simulink model "HIL_Testing_SW"  (Simulink 7.5)
settings: Solver=ode1  StartTime=0.0  StopTime=Inf  FixedStep=0.001  RelTol=1e-3
PostLoadFcn:
  | , if any(exist('dsrtsu_mdlpostloadfcn', 'file') == [2, 3, 6]), try dsrtsu_mdlpostloadfcn('Execute', bdroot); catch fprintf('Error in PostLoadFcn (dsrtsu_mdlpostloadfcn) for model "%s":\n %s\n', bdroot, lasterr); end, end,
undefined symbols (not defined in the file): CeBSER_Cnt_NumTempAxisPts, ChargeCord, ChargeCord_Control, ChargeToSOCCurr, ChrgCurrLim, CrntSens1Fine, CS_SOCSetPt, CyclerMaxChrgPwr, CyclerMaxDschrgPwr, deltaAhr, Drive_1, Drive_10, Drive_11, Drive_12, Drive_13, Drive_14, Drive_15, Drive_16, Drive_17, Drive_18, Drive_19, Drive_2, Drive_20, Drive_21, Drive_22, Drive_23, Drive_24, Drive_25, Drive_26, Drive_27, Drive_28, Drive_29, Drive_3, Drive_30, Drive_31, Drive_32, Drive_33, Drive_34, Drive_35, Drive_36, Drive_37, Drive_38, Drive_39, Drive_4, Drive_40, Drive_41, Drive_42, Drive_43, Drive_44, Drive_45, Drive_46, Drive_47, Drive_48, Drive_49, Drive_5, Drive_50, Drive_51, Drive_6, Drive_7, Drive_8 ... (+50)
libraries: simulink x129, rtican x50, rti2211sailib x5, rti2211serlib x5, rti2202miolib x3
(part 15 of 23)

== system HIL_Testing_SW/TX/Chiller/ChillerCmndTxDecision/ChillerCommands ==
  ReadChillerSP : Constant  Value=[82 83 13 13 13 13 13 13]  OutDataTypeMode=uint8  OutDataType=fixdt(1, 16)  OutScaling=2^0  OutDataTypeStr=uint8
  ReadChillerStatus : Constant  Value=[82 87 13 13 13 13 13 13]  OutDataTypeMode=uint8  OutDataType=fixdt(1, 16)  OutScaling=2^0  OutDataTypeStr=uint8
  ReadChillerTemp : Constant  Value=[82 84 13 13 13 13 13 13]  OutDataTypeMode=uint8  OutDataType=fixdt(1, 16)  OutScaling=2^0  OutDataTypeStr=uint8
  SetEchoOn : Constant  Value=[83 69 49 13 13 13 13 13]  OutDataTypeMode=uint8  OutDataType=fixdt(1, 16)  OutScaling=2^0  OutDataTypeStr=uint8
  TurnChillerOff : Constant  Value=[83 79 48 13 13 13 13 13]  OutDataTypeMode=uint8  OutDataType=fixdt(1, 16)  OutScaling=2^0  OutDataTypeStr=uint8
  TurnChillerOn : Constant  Value=[83 79 49 13 13 13 13 13]  OutDataTypeMode=uint8  OutDataType=fixdt(1, 16)  OutScaling=2^0  OutDataTypeStr=uint8
  TurnChiller_On : Outport
  TurnChiller_Off : Outport  Port=2
  SetEcho_On : Outport  Port=3
  ReadChiller_Status : Outport  Port=4
  ReadChillerSetPoint : Outport  Port=5
  ReadChiller_Temp : Outport  Port=6
  wires:
  TurnChillerOn/1 -> TurnChiller_On/1  "TurnChiller_On"
  TurnChillerOff/1 -> TurnChiller_Off/1  "TurnChiller_Off"
  SetEchoOn/1 -> SetEcho_On/1  "SetEcho_On"
  ReadChillerStatus/1 -> ReadChiller_Status/1  "ReadChiller_Status"
  ReadChillerSP/1 -> ReadChillerSetPoint/1  "ReadChillerSetPoint"
  ReadChillerTemp/1 -> ReadChiller_Temp/1  "ReadChiller_Temp"

== system HIL_Testing_SW/TX/Chiller/ChillerCmndTxDecision/ChillerRxProcessing ==
  RxBytes : Inport  OutDataType=fixdt(1, 16)  OutScaling=2^0
  NumRxBytes : Inport  Port=2  OutDataType=fixdt(1, 16)  OutScaling=2^0
  WaitRx : Inport  Port=3  OutDataType=fixdt(1, 16)  OutScaling=2^0
  ReadChillerStatus_Action : Inport  Port=4  OutDataType=fixdt(1, 16)  OutScaling=2^0
  ReadChillerSP_Action : Inport  Port=5  OutDataType=fixdt(1, 16)  OutScaling=2^0
  ReadChillerTemp_Action : Inport  Port=6  OutDataType=fixdt(1, 16)  OutScaling=2^0
  ChillerPositiveResponse : Subsystem
  ChillerStatus : Subsystem
  If : If  NumInputs=4  IfExpression=u1 == 1  ElseIfExpressions=u2 == 1, u3 == 1, u4 ==1
  ReadChillerSP : Subsystem  TreatAsAtomicUnit=on
  ReadChillerTemp : Subsystem
  RxChillerByteShifter : Subsystem
  Terminator : Terminator
  Terminator1 : Terminator
  Terminator2 : Terminator
  ChillerPosResponse : Outport  OutDataType=fixdt(1, 16)  OutScaling=2^0
  ChillerOn : Outport  Port=2  OutDataType=fixdt(1, 16)  OutScaling=2^0
  wires:
  RxBytes/1 -> RxChillerByteShifter/1(RxChillerBytes)
  ReadChillerSP/1(RxReadChillerSetPoint) -> Terminator/1
  ReadChillerTemp/1(RxReadChillerTemp) -> Terminator1/1
  If/1 -> ReadChillerSP/Action
  If/2 -> ReadChillerTemp/Action
  NumRxBytes/1 -> [NumRxBytes], RxChillerByteShifter/2(NumRxBytes)
  [NumRxBytes] -> ReadChillerSP/1(NumRxBytes)
  [NumRxBytes] -> ReadChillerTemp/1(NumRxBytes)
  If/5 -> Terminator2/1
  ChillerPositiveResponse/1(ChillerPositiveResponse) -> ChillerPosResponse/1
  WaitRx/1 -> If/3
  ReadChillerStatus_Action/1 -> If/4
  If/4 -> ChillerStatus/Action
  ChillerStatus/1(ChillerOn) -> ChillerOn/1
  If/3 -> ChillerPositiveResponse/Action
  ReadChillerTemp_Action/1 -> If/2
  ReadChillerSP_Action/1 -> If/1

== system HIL_Testing_SW/TX/Chiller/ChillerCmndTxDecision/CreateChillerSPCmnd ==
  ChillerT_SP : Inport  OutDataType=fixdt(1, 16)  OutScaling=2^0
  ChillerMux : Mux  Inputs=8
      settings: DisplayOption=signals
  DeMuxChillerInputNumber : Subsystem
  SetChillerSPCmnd : Outport  OutDataType=fixdt(1, 16)  OutScaling=2^0
  wires:
  ChillerT_SP/1 -> DeMuxChillerInputNumber/1(ChillerSP_Number)
  DeMuxChillerInputNumber/4(OnesDigitAscii) -> ChillerMux/5
  DeMuxChillerInputNumber/6(TenthsDigitAscii) -> ChillerMux/7
  ChillerMux/1 -> SetChillerSPCmnd/1
  DeMuxChillerInputNumber/2(PosOrNegAscii) -> ChillerMux/3
  DeMuxChillerInputNumber/3(TensDigitAscii) -> ChillerMux/4
  DeMuxChillerInputNumber/1(Ascii_S) -> ChillerMux/1, ChillerMux/2
  DeMuxChillerInputNumber/5(Ascii_Pt) -> ChillerMux/6
  DeMuxChillerInputNumber/7(Ascii_CarriageReturn) -> ChillerMux/8

== system HIL_Testing_SW/TX/Chiller/ChillerCmndTxDecision/CreateChillerSPCmnd2 ==
  ChillerT_SP : Inport  OutDataType=fixdt(1, 16)  OutScaling=2^0
  ChillerMux : Mux  Inputs=8
      settings: DisplayOption=signals
  DeMuxChillerInputNumber : Subsystem
  Gain : Gain  ParameterDataType=fixdt(1, 16)  ParameterScaling=2^0  OutDataTypeMode=uint8  OutDataType=fixdt(1, 16)  OutScaling=2^0  OutDataTypeStr=uint8
  SetChillerSPCmnd : Outport  OutDataType=fixdt(1, 16)  OutScaling=2^0
  wires:
  DeMuxChillerInputNumber/7(Ascii_CarriageReturn) -> ChillerMux/8
  DeMuxChillerInputNumber/5(Ascii_Pt) -> ChillerMux/6
  DeMuxChillerInputNumber/1(Ascii_S) -> ChillerMux/2, ChillerMux/1
  DeMuxChillerInputNumber/3(TensDigitAscii) -> ChillerMux/4
  DeMuxChillerInputNumber/2(PosOrNegAscii) -> ChillerMux/3
  ChillerMux/1 -> Gain/1
  DeMuxChillerInputNumber/6(TenthsDigitAscii) -> ChillerMux/7
  DeMuxChillerInputNumber/4(OnesDigitAscii) -> ChillerMux/5
  ChillerT_SP/1 -> DeMuxChillerInputNumber/1(ChillerSP_Number)
  Gain/1 -> SetChillerSPCmnd/1

== system HIL_Testing_SW/TX/TX PTEI/Tx_Contactor_Msg/msg_0x186 ==
  Ignition : Inport  OutDataType=fixdt(1, 16)  OutScaling=2^0
  InvVoltatge : Inport  Port=2  OutDataType=fixdt(1, 16)  OutScaling=2^0
  Trigger : TriggerPort  TriggerType=function-call
  ContactorsClosed1 : Constant  OutDataType=sfix(16)  OutScaling=2^0  OutDataTypeStr=Inherit: Inherit via back propagation
  ContactorsClosed4 : Constant  Value=0  OutDataType=sfix(16)  OutScaling=2^0  OutDataTypeStr=Inherit: Inherit via back propagation
  Ground_{1..16} (16 alike) : Ground
  PTEI_Hybrid_Status_1 : rtican/RTICAN Transmit (TX)   SystemSampleTime=-1  Reserved1=[]  Reserved2=[]  Reserved3=[]  Reserved4=[]  SfcnMessage=[]  Msg_Struct=[]  BoardTypeNo=[]  BoardNo=[]  ChannelNo=[]  Parameters=[]  DialogFcn=[]  UnitName=[]  Revision=[]  UnitValues=[]  DSProperties=struct('RTI',struct('Version',uint32(5),'BlockType',struct('isSLSource',uint8(1),'isSLSink',uint8(1),'isHWSource',uint8(0),'isHWSink',uint8(0),'isSetup',uint8(0),'isInline',uint8(1),'isNonInline',uint8(0),'isInterrupt',uint8(0),'isChannelwise',uint8(0)),'IOBoardType','RTICAN','UnitType','MESSAGE','Identifier','TX','DialogType','MSVC','BlockSet','RTICAN','SlaveProcessor','CAN'))  RTIBlockInterface=struct('InputPortsWidth',int32([1 1 1 1 1 1 1 1 1 1 1 1 1 1 1 1 1 1 1]),'InputPortsActive',[1 1 1 1 1 1 1 1 1 1 1 1 1 1 1 1 1 1 1],'InputPortsName',{{'RdHVInvRatVlt','HybCrpCstCrvRq','EstMtrPwrLoss','HybGrdBrkgAct','TransFldPmpMtrDrtd','EngActDmpgDsblReq','HybACCompRq','EstMtrPwrLossV','HybExtndDcFuelCORq','HybCmmdEngTrqLmtd','HESSI_EngStrtTyp','HESSI_EngStrtStpMd','HybCrnkAbrtd','CnvntlEngStrtEnbld','RdPTHVCntrReq','HybCmmFailRdPwrCmd','HybRdcdTrqCapMd1Cmnd','HybDFCOReq','RdHVInvRatVltV'}},'InputPortsDataType',{{'SS_DOUBLE','SS_DOUBLE','SS_DOUBLE','SS_DOUBLE','SS_DOUBLE','SS_DOUBLE','SS_DOUBLE','SS_DOUBLE','SS_DOUBLE','SS_DOUBLE','SS_DOUBLE','SS_DOUBLE','SS_DOUBLE','SS_DOUBLE','SS_DOUBLE','SS_DOUBLE','SS_DOUBLE','SS_DOUBLE','SS_DOUBLE'}},'OutputPortsWidth',int32(0),'OutputPortsActive',0,'OutputPortsName',{{''}},'DialogFcn','rtican_message_interface_gui','BlockDisplay',{{'','center'}},'IconTransparency','on','InitLevel',3,'BlockName',struct('Token',{{'PTEI_Hybrid_Status_1'}}),'SampleTime',{{-1}},'TriggerPort',{{'none'}},'EnablePort',{{'none'}})  RTIBlockParameters=struct('BoardTypeNo',{{4302,'OFF',[]}},'BoardNo',{{1,'ON',[1 16]}},'ChannelNo',{{1,'ON',[1 4]}},'Parameters',{{struct('DataFileSupport',struct('DataFileSelectedMaster',1,'DataFileSelectedLocal',1,'DataFileName',['c:\data\databases\8.4.5 (140425)\globala - hs.dbc|'],'DataFileDate',{{{['24-Apr-2014 15:37:04']}}},'SelectedFile',['..\databases\8.4.5 (140425)\globala - hs.dbc'],'InterfaceFcn','rtican_dbc_file_parser'),'Options',struct('StatusSelected',0,'TimeSelected',0,'DeltaTimeSelected',0,'DelayTimeSelected',0,'DelayTimeTXCommandSelected',0,'EncodeSetUnusedBitsToOne',0,'EnableMsgLoopback',0,'TriggerPort',struct('Selected',0,'TriggerType',0),'EnablePortSelected',0,'SignalOnPortnameSelected',1,'UserCoding',struct('Selected',0,'InterfaceFile','UserEncodingFile','FcnName','UserEncodeFcn','InportSelected',0,'InportWidth',1,'OutportSelected',0,'OutportWidth',1),'TerminationMsg',struct('Selected',0,'Byte0_7','0'),'InitialMsg',struct('Selected',0,'Byte0_7','0')),'Message',struct('MsgOnBlocknameSelected',1,'MsgName','PTEI_Hybrid_Status_1','MsgIdFormat',0,'MsgId',390,'MsgLength',7,'NumSignals',19,'SampleTime',-1,'StartTime',struct('Selected',0,'Value',0),'AutoRepeatTime',struct('Selected',0,'Value',0.1),'Timeout',struct('Selected',0,'Value',0.1),'DelayTime',struct('Selected',0,'Value',0.1),'Signal',struct('SgnName',{'RdHVInvRatVlt','HybCrpCstCrvRq','EstMtrPwrLoss','HybGrdBrkgAct','TransFldPmpMtrDrtd','EngActDmpgDsblReq','HybACCompRq','EstMtrPwrLossV','HybExtndDcFuelCORq','HybCmmdEngTrqLmtd','HESSI_EngStrtTyp','HESSI_EngStrtStpMd','HybCrnkAbrtd','CnvntlEngStrtEnbld','RdPTHVCntrReq','HybCmmFailRdPwrCmd','HybRdcdTrqCapMd1Cmnd','HybDFCOReq','RdHVInvRatVltV'},'SgnStartBit',{0,9,16,25,26,27,28,30,31,32,40,44,48,49,50,52,53,54,55},'SgnLength',{9,3,8,1,1,1,2,1,1,8,4,4,1,1,2,1,1,1,1},'SgnType',{0,0,0,0,0,0,0,0,0,0,0,0,0,0,0,0,0,0,0},'ModeValue',{-1,-1,-1,-1,-1,-1,-1,-1,-1,-1,-1,-1,-1,-1,-1,-1,-1,-1,-1},'DataType',{0,0,0,0,0,0,0,0,0,0,0,0,0,0,0,0,0,0,0},'ByteLayout',{2,2,2,2,2,2,2,2,2,2,2,2,2,2,2,2,2,2,2},'Factor',{1,1,0.25,1,1,1,1,1,1,0.75,1,1,1,1,1,1,1,1,1},'Offset',{0,0,0,0,0,0,0,0,0,-90,0,0,0,0,0,0,0,0,0},'SgnComment',{{''},{''},{''},{''},{''},{''},{''},{''},{''},{''},{''},{''},{''},{''},{''},{''},{''},{['DFCO = Deceleration Fuel Cut Off']},{''}},'SgnUnit',{'volts','','kW','','','','','','','Nm','','','','','','','','',''},'Min',{0,0,0,0,0,0,0,0,0,-90,0,0,0,0,0,0,0,0,0},'Max',{511,7,63.75,1,1,1,3,1,1,101.25,15,15,1,1,3,1,1,1,1},'SLDataType',{'SS_DOUBLE','SS_DOUBLE','SS_DOUBLE','SS_DOUBLE','SS_DOUBLE','SS_DOUBLE','SS_DOUBLE','SS_DOUBLE','SS_DOUBLE','SS_DOUBLE','SS_DOUBLE','SS_DOUBLE','SS_DOUBLE','SS_DOUBLE','SS_DOUBLE','SS_DOUBLE','SS_DOUBLE','SS_DOUBLE','SS_DOUBLE'}),'MsgIdNumFormat',0,'MsgComment',{{''}}),'Version',1.2,'general',struct('isFromLib',0)),'OFF',[]}},'GroupId',{{struct('Group',{{'RTICAN'}},'No',8,'Behavior',{{'NAMECHANGE'}},'BlockType',{{'SINK'}},'NameChangeFlag',0),'OFF',[]}},'SFcnRTICANMessage',{{struct('MsgType','TX','SFcnPortType','Scalar','MsgName','PTEI_Hybrid_Status_1','MsgIdFormat','STD','MsgId',390,'MsgLength',7,'NumSignals',19,'SampleTime',-1,'StartTime',struct('Selected','no','Value',0),'AutoRepeatTime',struct('Selected','no','Value',0.1),'Timeout',struct('Selected','no','Value',0.1),'Signal',struct('SgnName',{'RdHVInvRatVlt','HybCrpCstCrvRq','EstMtrPwrLoss','HybGrdBrkgAct','TransFldPmpMtrDrtd','EngActDmpgDsblReq','HybACCompRq','EstMtrPwrLossV','HybExtndDcFuelCORq','HybCmmdEngTrqLmtd','HESSI_EngStrtTyp','HESSI_EngStrtStpMd','HybCrnkAbrtd','CnvntlEngStrtEnbld','RdPTHVCntrReq','HybCmmFailRdPwrCmd','HybRdcdTrqCapMd1Cmnd','HybDFCOReq','RdHVInvRatVltV'},'SgnStartBit',{0,9,16,25,26,27,28,30,31,32,40,44,48,49,50,52,53,54,55},'SgnLength',{9,3,8,1,1,1,2,1,1,8,4,4,1,1,2,1,1,1,1},'SgnType',{'standard','standard','standard','standard','standard','standard','standard','standard','standard','standard','standard','standard','standard','standard','standard','standard','standard','standard','standard'},'ModeValue',{-1,-1,-1,-1,-1,-1,-1,-1,-1,-1,-1,-1,-1,-1,-1,-1,-1,-1,-1},'DataType',{['unsigned int'],['unsigned int'],['unsigned int'],['unsigned int'],['unsigned int'],['unsigned int'],['unsigned int'],['unsigned int'],['unsigned int'],['unsigned int'],['unsigned int'],['unsigned int'],['unsigned int'],['unsigned int'],['unsigned int'],['unsigned int'],['unsigned int'],['unsigned int'],['unsigned int']},'ByteLayout',{['motorola back.'],['motorola back.'],['motorola back.'],['motorola back.'],['motorola back.'],['motorola back.'],['motorola back.'],['motorola back.'],['motorola back.'],['motorola back.'],['motorola back.'],['motorola back.'],['motorola back.'],['motorola back.'],['motorola back.'],['motorola back.'],['motorola back.'],['motorola back.'],['motorola back.']},'Factor',{1,1,0.25,1,1,1,1,1,1,0.75,1,1,1,1,1,1,1,1,1},'Offset',{0,0,0,0,0,0,0,0,0,-90,0,0,0,0,0,0,0,0,0},'SLDataType',{'SS_DOUBLE','SS_DOUBLE','SS_DOUBLE','SS_DOUBLE','SS_DOUBLE','SS_DOUBLE','SS_DOUBLE','SS_DOUBLE','SS_DOUBLE','SS_DOUBLE','SS_DOUBLE','SS_DOUBLE','SS_DOUBLE','SS_DOUBLE','SS_DOUBLE','SS_DOUBLE','SS_DOUBLE','SS_DOUBLE','SS_DOUBLE'}),'StatusSelected','no','TimeSelected','no','DeltaTimeSelected','no','DelayTimeSelected','no','DelayTimeTXCommandSelected','no','EncodeSetUnusedBitsToOne','no','EnableMsgLoopback','no','TriggerPort',struct('Selected','no','TriggerType',0),'EnablePortSelected','no','UserCoding',struct('Selected','no','InterfaceFile','UserEncodingFile','FcnName','UserEncodeFcn','InportSelected','no','InportWidth',1,'OutportSelected','no','OutportWidth',1),'TerminationMsg',struct('Selected','no','Byte0','0x00','Byte1','0x00','Byte2','0x00','Byte3','0x00','Byte4','0x00','Byte5','0x00','Byte6','0x00','Byte7','0x00'),'InitialMsg',struct('Selected','no','Byte0','0x00','Byte1','0x00','Byte2','0x00','Byte3','0x00','Byte4','0x00','Byte5','0x00','Byte6','0x00','Byte7','0x00'),'BoardType','DS4302','BoardNo',1,'ControllerNo',1),'OFF',[]}},'TLCFileName',{{'rtican_tx_message','OFF',[]}})  RTISFcnParameters=struct('SFcnRTICANMessage','struct','TLCFileName','char')  RTIBlockParaDefault=struct('BoardTypeNo',4302,'BoardNo',1,'ChannelNo',1,'Parameters',struct('DataFileSupport',struct('DataFileSelectedMaster',0,'DataFileSelectedLocal',0,'DataFileName','','DataFileDate','','SelectedFile',['<no file selected>']),'Options',struct('StatusSelected',1,'TimeSelected',1,'DeltaTimeSelected',1,'DelayTimeSelected',1,'DelayTimeTXCommandSelected',0,'EncodeSetUnusedBitsToOne',0,'EnableMsgLoopback',0,'TriggerPort',struct('Selected',0,'TriggerType','rising'),'EnablePortSelected',0,'SignalOnPortnameSelected',1,'UserCoding',struct('Selected',0,'InterfaceFile','UserEncodingFile','FcnName','UserEncodeFcn','InportSelected',0,'InportWidth',1,'OutportSelected',0,'OutportWidth',1),'TerminationMsg',struct('Selected',0,'Byte0_7','0'),'InitialMsg',struct('Selected',0,'Byte0_7','0')),'Message',struct('MsgOnBlocknameSelected',0,'MsgName',['TX Message'],'MsgIdFormat',0,'MsgId',100,'MsgLength',8,'NumSignals',1,'SampleTime',-1,'StartTime',struct('Selected',0,'Value',0),'AutoRepeatTime',struct('Selected',0,'Value',0.1),'Timeout',struct('Selected',0,'Value',0.1),'DelayTime',struct('Selected',0,'Value',0.1),'Signal',struct('SgnName',['TX signal'],'SgnStartBit',0,'SgnLength',8,'SgnType',0,'ModeValue',-1,'DataType',0,'SLDataType','SS_DOUBLE','ByteLayout',0,'Factor',1,'Offset',0,'Min',0,'Max',255,'SgnComment',{{}},'SgnUnit',''),'MsgIdNumFormat',0,'MsgComment',{{''}}),'Version',1.2,'general',struct('isFromLib',1)),'GroupId',struct('Group',{{'RTICAN'}},'No',1,'Behavior',{{'NAMECHANGE'}},'BlockType',{{'SINK'}},'NameChangeFlag',0),'SFcnRTICANMessage',struct('MsgType','TX','MsgName',['TX Message'],'MsgIdFormat','STD','MsgId',100,'MsgLength',2,'NumSignals',1,'SampleTime',-1,'StartTime',struct('Selected','no','Value',0),'AutoRepeatTime',struct('Selected','no','Value',0.1),'Timeout',struct('Selected','no','Value',0.1),'DelayTime',struct('Selected','no','Value',0.1),'Signal',struct('SgnName',['TX signal'],'SgnStartBit',0,'SgnLength',8,'SgnType','standard','ModeValue',-1,'DataType',['unsigned int'],'ByteLayout',['little endian'],'SLDataType','SS_DOUBLE','Factor',1,'Offset',0),'StatusSelected','yes','TimeSelected','yes','DeltaTimeSelected','yes','DelayTimeSelected','yes','EnablePortSelected','no','EnableMsgLoopback','no','DelayTimeTXCommandSelected','no','EncodeSetUnusedBitsToOne','no','UserCoding',struct('Selected','no','InterfaceFile','UserDecodingFile','FcnName','UserDecodeFcn','InportSelected','no','InportWidth',1,'OutportSelected','no','OutportWidth',1),'TerminationMsg',struct('Selected','no','Byte0','0x00','Byte1','0x00','Byte2','0x00','Byte3','0x00','Byte4','0x00','Byte5','0x00','Byte6','0x00','Byte7','0x00'),'InitialMsg',struct('Selected','no','Byte0','0x00','Byte1','0x00','Byte2','0x00','Byte3','0x00','Byte4','0x00','Byte5','0x00','Byte6','0x00','Byte7','0x00'),'TriggerPort',struct('Selected','no','TriggerType','rising'),'BoardType','DS4302','BoardNo',1,'ControllerNo',1,'SFcnPortType','Scalar'),'TLCFileName','rtican_tx_message')
      settings: AttributesFormatString=Group Id: RTICAN8\n
  Switch : Switch  Threshold=0.5  OutDataType=fixdt(1, 16)  OutScaling=2^0  OutDataTypeStr=Inherit: Inherit via back propagation
  validity : Constant  Value=0  OutDataType=sfix(16)  OutScaling=2^0  OutDataTypeStr=Inherit: Inherit via back propagation
  wires:
  InvVoltatge/1 -> PTEI_Hybrid_Status_1/1
  validity/1 -> PTEI_Hybrid_Status_1/19
  ContactorsClosed1/1 -> Switch/1
  Ignition/1 -> Switch/2
  ContactorsClosed4/1 -> Switch/3
  Switch/1 -> PTEI_Hybrid_Status_1/15
  Ground_1/1 -> PTEI_Hybrid_Status_1/3
  Ground_2/1 -> PTEI_Hybrid_Status_1/6
  Ground_3/1 -> PTEI_Hybrid_Status_1/7
  Ground_4/1 -> PTEI_Hybrid_Status_1/8
  Ground_5/1 -> PTEI_Hybrid_Status_1/9
  Ground_6/1 -> PTEI_Hybrid_Status_1/10
  Ground_7/1 -> PTEI_Hybrid_Status_1/11
  Ground_8/1 -> PTEI_Hybrid_Status_1/12
  Ground_9/1 -> PTEI_Hybrid_Status_1/13
  Ground_10/1 -> PTEI_Hybrid_Status_1/14
  Ground_11/1 -> PTEI_Hybrid_Status_1/16
  Ground_13/1 -> PTEI_Hybrid_Status_1/18
  Ground_14/1 -> PTEI_Hybrid_Status_1/2
  Ground_15/1 -> PTEI_Hybrid_Status_1/4
  Ground_12/1 -> PTEI_Hybrid_Status_1/17
  Ground_16/1 -> PTEI_Hybrid_Status_1/5

== system HIL_Testing_SW/TX/TX PTEI/Tx_Contactor_Msg/msg_0x1E3 ==
  HVInvRatVlt : Inport  OutDataType=sfix(16)  OutScaling=2^0
  Trigger : TriggerPort  TriggerType=function-call
  Constant{,1..10,12..13} (13 alike) : Constant  Value=0  OutDataType=sfix(16)  OutScaling=2^0
  Data Type Conversion{1..14} (14 alike) : DataTypeConversion  OutDataType=fixdt(1, 16)  OutScaling=2^0
  PPEI_Hybrid_High_Voltage_Status : rtican/RTICAN Transmit (TX)   SystemSampleTime=-1  Reserved1=[]  Reserved2=[]  Reserved3=[]  Reserved4=[]  SfcnMessage=[]  Msg_Struct=[]  BoardTypeNo=[]  BoardNo=[]  ChannelNo=[]  Parameters=[]  DialogFcn=[]  UnitName=[]  Revision=[]  UnitValues=[]  DSProperties=struct('RTI',struct('Version',uint32(5),'BlockType',struct('isSLSource',uint8(1),'isSLSink',uint8(1),'isHWSource',uint8(0),'isHWSink',uint8(0),'isSetup',uint8(0),'isInline',uint8(1),'isNonInline',uint8(0),'isInterrupt',uint8(0),'isChannelwise',uint8(0)),'IOBoardType','RTICAN','UnitType','MESSAGE','Identifier','TX','DialogType','MSVC','BlockSet','RTICAN','SlaveProcessor','CAN'))  RTIBlockInterface=struct('InputPortsWidth',int32([1 1 1 1 1 1 1 1 1 1 1 1 1 1]),'InputPortsActive',[1 1 1 1 1 1 1 1 1 1 1 1 1 1],'InputPortsName',{{'AccPowModPowUsd','PTBatRsrvPwrReq','HybSysNonEmissRMAct','JmpStrtEnbldStat','PwrElecCoolPmpReq','HybEngReqOn','HybNEmsRltMalfActv','HybChrgMdStat','HVInvRatVlt','HVInvRatVltV','PTHVCShdwnCmplt','PTHVCntctrReq','HVPsvIsStat','HVActDisCmnd'}},'InputPortsDataType',{{'SS_DOUBLE','SS_DOUBLE','SS_DOUBLE','SS_DOUBLE','SS_DOUBLE','SS_DOUBLE','SS_DOUBLE','SS_DOUBLE','SS_DOUBLE','SS_DOUBLE','SS_DOUBLE','SS_DOUBLE','SS_DOUBLE','SS_DOUBLE'}},'OutputPortsWidth',int32(1),'OutputPortsActive',1,'OutputPortsName',{{['TX status']}},'DialogFcn','rtican_message_interface_gui','BlockDisplay',{{'','center'}},'IconTransparency','on','InitLevel',3,'BlockName',struct('Token',{{'PPEI_Hybrid_High_Voltage_Status'}}),'SampleTime',{{-1}},'TriggerPort',{{'none'}},'EnablePort',{{'none'}})  RTIBlockParameters=struct('BoardTypeNo',{{4302,'OFF',[]}},'BoardNo',{{1,'ON',[1 16]}},'ChannelNo',{{2,'ON',[1 4]}},'Parameters',{{struct('DataFileSupport',struct('DataFileSelectedMaster',1,'DataFileSelectedLocal',1,'DataFileName',['c:\data\databases\8.4.5 (140425)\globala - pe.dbc|'],'DataFileDate',{{{['24-Apr-2014 15:33:48']}}},'SelectedFile',['..\databases\8.4.5 (140425)\globala - pe.dbc'],'InterfaceFcn','rtican_dbc_file_parser'),'Options',struct('StatusSelected',1,'TimeSelected',0,'DeltaTimeSelected',0,'DelayTimeSelected',0,'DelayTimeTXCommandSelected',0,'EncodeSetUnusedBitsToOne',0,'EnableMsgLoopback',0,'TriggerPort',struct('Selected',0,'TriggerType',0),'EnablePortSelected',0,'SignalOnPortnameSelected',1,'UserCoding',struct('Selected',0,'InterfaceFile','UserEncodingFile','FcnName','UserEncodeFcn','InportSelected',0,'InportWidth',1,'OutportSelected',0,'OutportWidth',1),'TerminationMsg',struct('Selected',0,'Byte0_7','0'),'InitialMsg',struct('Selected',0,'Byte0_7','0')),'Message',struct('MsgOnBlocknameSelected',1,'MsgName','PPEI_Hybrid_High_Voltage_Status','MsgIdFormat',0,'MsgId',483,'MsgLength',7,'NumSignals',14,'SampleTime',-1,'StartTime',struct('Selected',0,'Value',0),'AutoRepeatTime',struct('Selected',0,'Value',0.1),'Timeout',struct('Selected',0,'Value',0.1),'DelayTime',struct('Selected',0,'Value',0.1),'Signal',struct('SgnName',{'AccPowModPowUsd','PTBatRsrvPwrReq','HybSysNonEmissRMAct','JmpStrtEnbldStat','PwrElecCoolPmpReq','HybEngReqOn','HybNEmsRltMalfActv','HybChrgMdStat','HVInvRatVlt','HVInvRatVltV','PTHVCShdwnCmplt','PTHVCntctrReq','HVPsvIsStat','HVActDisCmnd'},'SgnStartBit',{0,24,28,29,32,35,36,38,40,49,50,51,53,55},'SgnLength',{9,2,1,3,2,1,1,2,9,1,1,2,2,1},'SgnType',{0,0,0,0,0,0,0,0,0,0,0,0,0,0},'ModeValue',{-1,-1,-1,-1,-1,-1,-1,-1,-1,-1,-1,-1,-1,-1},'DataType',{0,0,0,0,0,0,0,0,0,0,0,0,0,0},'ByteLayout',{2,2,2,2,2,2,2,2,2,2,2,2,2,2},'Factor',{0.01,1,1,1,1,1,1,1,1,1,1,1,1,1},'Offset',{0,0,0,0,0,0,0,0,0,0,0,0,0,0},'SgnComment',{{''},{''},{''},{''},{''},{''},{''},{''},{''},{''},{''},{''},{''},{''}},'SgnUnit',{'kW','','','','','','','','volts','','','','',''},'Min',{0,0,0,0,0,0,0,0,0,0,0,0,0,0},'Max',{5.11,3,1,7,3,1,1,3,511,1,1,3,3,1},'SLDataType',{'SS_DOUBLE','SS_DOUBLE','SS_DOUBLE','SS_DOUBLE','SS_DOUBLE','SS_DOUBLE','SS_DOUBLE','SS_DOUBLE','SS_DOUBLE','SS_DOUBLE','SS_DOUBLE','SS_DOUBLE','SS_DOUBLE','SS_DOUBLE'}),'MsgIdNumFormat',0,'MsgComment',{{''}}),'Version',1.2,'general',struct('isFromLib',0)),'OFF',[]}},'GroupId',{{struct('Group',{{'RTICAN'}},'No',5,'Behavior',{{'NAMECHANGE'}},'BlockType',{{'SINK'}},'NameChangeFlag',0),'OFF',[]}},'SFcnRTICANMessage',{{struct('MsgType','TX','SFcnPortType','Scalar','MsgName','PPEI_Hybrid_High_Voltage_Status','MsgIdFormat','STD','MsgId',483,'MsgLength',7,'NumSignals',14,'SampleTime',-1,'StartTime',struct('Selected','no','Value',0),'AutoRepeatTime',struct('Selected','no','Value',0.1),'Timeout',struct('Selected','no','Value',0.1),'Signal',struct('SgnName',{'AccPowModPowUsd','PTBatRsrvPwrReq','HybSysNonEmissRMAct','JmpStrtEnbldStat','PwrElecCoolPmpReq','HybEngReqOn','HybNEmsRltMalfActv','HybChrgMdStat','HVInvRatVlt','HVInvRatVltV','PTHVCShdwnCmplt','PTHVCntctrReq','HVPsvIsStat','HVActDisCmnd'},'SgnStartBit',{0,24,28,29,32,35,36,38,40,49,50,51,53,55},'SgnLength',{9,2,1,3,2,1,1,2,9,1,1,2,2,1},'SgnType',{'standard','standard','standard','standard','standard','standard','standard','standard','standard','standard','standard','standard','standard','standard'},'ModeValue',{-1,-1,-1,-1,-1,-1,-1,-1,-1,-1,-1,-1,-1,-1},'DataType',{['unsigned int'],['unsigned int'],['unsigned int'],['unsigned int'],['unsigned int'],['unsigned int'],['unsigned int'],['unsigned int'],['unsigned int'],['unsigned int'],['unsigned int'],['unsigned int'],['unsigned int'],['unsigned int']},'ByteLayout',{['motorola back.'],['motorola back.'],['motorola back.'],['motorola back.'],['motorola back.'],['motorola back.'],['motorola back.'],['motorola back.'],['motorola back.'],['motorola back.'],['motorola back.'],['motorola back.'],['motorola back.'],['motorola back.']},'Factor',{0.01,1,1,1,1,1,1,1,1,1,1,1,1,1},'Offset',{0,0,0,0,0,0,0,0,0,0,0,0,0,0},'SLDataType',{'SS_DOUBLE','SS_DOUBLE','SS_DOUBLE','SS_DOUBLE','SS_DOUBLE','SS_DOUBLE','SS_DOUBLE','SS_DOUBLE','SS_DOUBLE','SS_DOUBLE','SS_DOUBLE','SS_DOUBLE','SS_DOUBLE','SS_DOUBLE'}),'StatusSelected','yes','TimeSelected','no','DeltaTimeSelected','no','DelayTimeSelected','no','DelayTimeTXCommandSelected','no','EncodeSetUnusedBitsToOne','no','EnableMsgLoopback','no','TriggerPort',struct('Selected','no','TriggerType',0),'EnablePortSelected','no','UserCoding',struct('Selected','no','InterfaceFile','UserEncodingFile','FcnName','UserEncodeFcn','InportSelected','no','InportWidth',1,'OutportSelected','no','OutportWidth',1),'TerminationMsg',struct('Selected','no','Byte0','0x00','Byte1','0x00','Byte2','0x00','Byte3','0x00','Byte4','0x00','Byte5','0x00','Byte6','0x00','Byte7','0x00'),'InitialMsg',struct('Selected','no','Byte0','0x00','Byte1','0x00','Byte2','0x00','Byte3','0x00','Byte4','0x00','Byte5','0x00','Byte6','0x00','Byte7','0x00'),'BoardType','DS4302','BoardNo',1,'ControllerNo',2),'OFF',[]}},'TLCFileName',{{'rtican_tx_message','OFF',[]}})  RTISFcnParameters=struct('SFcnRTICANMessage','struct','TLCFileName','char')  RTIBlockParaDefault=struct('BoardTypeNo',4302,'BoardNo',1,'ChannelNo',1,'Parameters',struct('DataFileSupport',struct('DataFileSelectedMaster',0,'DataFileSelectedLocal',0,'DataFileName','','DataFileDate','','SelectedFile',['<no file selected>']),'Options',struct('StatusSelected',1,'TimeSelected',1,'DeltaTimeSelected',1,'DelayTimeSelected',1,'DelayTimeTXCommandSelected',0,'EncodeSetUnusedBitsToOne',0,'EnableMsgLoopback',0,'TriggerPort',struct('Selected',0,'TriggerType','rising'),'EnablePortSelected',0,'SignalOnPortnameSelected',1,'UserCoding',struct('Selected',0,'InterfaceFile','UserEncodingFile','FcnName','UserEncodeFcn','InportSelected',0,'InportWidth',1,'OutportSelected',0,'OutportWidth',1),'TerminationMsg',struct('Selected',0,'Byte0_7','0'),'InitialMsg',struct('Selected',0,'Byte0_7','0')),'Message',struct('MsgOnBlocknameSelected',0,'MsgName',['TX Message'],'MsgIdFormat',0,'MsgId',100,'MsgLength',8,'NumSignals',1,'SampleTime',-1,'StartTime',struct('Selected',0,'Value',0),'AutoRepeatTime',struct('Selected',0,'Value',0.1),'Timeout',struct('Selected',0,'Value',0.1),'DelayTime',struct('Selected',0,'Value',0.1),'Signal',struct('SgnName',['TX signal'],'SgnStartBit',0,'SgnLength',8,'SgnType',0,'ModeValue',-1,'DataType',0,'SLDataType','SS_DOUBLE','ByteLayout',0,'Factor',1,'Offset',0,'Min',0,'Max',255,'SgnComment',{{}},'SgnUnit',''),'MsgIdNumFormat',0,'MsgComment',{{''}}),'Version',1.2,'general',struct('isFromLib',1)),'GroupId',struct('Group',{{'RTICAN'}},'No',1,'Behavior',{{'NAMECHANGE'}},'BlockType',{{'SINK'}},'NameChangeFlag',0),'SFcnRTICANMessage',struct('MsgType','TX','MsgName',['TX Message'],'MsgIdFormat','STD','MsgId',100,'MsgLength',2,'NumSignals',1,'SampleTime',-1,'StartTime',struct('Selected','no','Value',0),'AutoRepeatTime',struct('Selected','no','Value',0.1),'Timeout',struct('Selected','no','Value',0.1),'DelayTime',struct('Selected','no','Value',0.1),'Signal',struct('SgnName',['TX signal'],'SgnStartBit',0,'SgnLength',8,'SgnType','standard','ModeValue',-1,'DataType',['unsigned int'],'ByteLayout',['little endian'],'SLDataType','SS_DOUBLE','Factor',1,'Offset',0),'StatusSelected','yes','TimeSelected','yes','DeltaTimeSelected','yes','DelayTimeSelected','yes','EnablePortSelected','no','EnableMsgLoopback','no','DelayTimeTXCommandSelected','no','EncodeSetUnusedBitsToOne','no','UserCoding',struct('Selected','no','InterfaceFile','UserDecodingFile','FcnName','UserDecodeFcn','InportSelected','no','InportWidth',1,'OutportSelected','no','OutportWidth',1),'TerminationMsg',struct('Selected','no','Byte0','0x00','Byte1','0x00','Byte2','0x00','Byte3','0x00','Byte4','0x00','Byte5','0x00','Byte6','0x00','Byte7','0x00'),'InitialMsg',struct('Selected','no','Byte0','0x00','Byte1','0x00','Byte2','0x00','Byte3','0x00','Byte4','0x00','Byte5','0x00','Byte6','0x00','Byte7','0x00'),'TriggerPort',struct('Selected','no','TriggerType','rising'),'BoardType','DS4302','BoardNo',1,'ControllerNo',1,'SFcnPortType','Scalar'),'TLCFileName','rtican_tx_message')
      settings: AttributesFormatString=Group Id: RTICAN5\n
  PTHVCntctrReq : Constant  OutDataType=sfix(16)  OutScaling=2^0
  Terminator : Terminator
  wires:
  PPEI_Hybrid_High_Voltage_Status/1 -> Terminator/1
  Constant/1 -> PPEI_Hybrid_High_Voltage_Status/1
  Constant1/1 -> Data Type Conversion1/1
  Constant2/1 -> Data Type Conversion3/1
  Constant3/1 -> Data Type Conversion4/1
  Constant4/1 -> Data Type Conversion5/1
  Constant5/1 -> Data Type Conversion7/1
  Constant7/1 -> Data Type Conversion8/1
  Constant6/1 -> Data Type Conversion9/1
  PTHVCntctrReq/1 -> Data Type Conversion10/1
  Constant9/1 -> Data Type Conversion11/1
  Constant8/1 -> Data Type Conversion12/1
  HVInvRatVlt/1 -> Data Type Conversion13/1
  Constant12/1 -> Data Type Conversion6/1
  Constant13/1 -> Data Type Conversion2/1
  Data Type Conversion13/1 -> PPEI_Hybrid_High_Voltage_Status/9
  Data Type Conversion2/1 -> PPEI_Hybrid_High_Voltage_Status/2
  Data Type Conversion3/1 -> PPEI_Hybrid_High_Voltage_Status/5
  Data Type Conversion5/1 -> PPEI_Hybrid_High_Voltage_Status/6
  Data Type Conversion6/1 -> PPEI_Hybrid_High_Voltage_Status/7
  Data Type Conversion7/1 -> PPEI_Hybrid_High_Voltage_Status/8
  Data Type Conversion8/1 -> PPEI_Hybrid_High_Voltage_Status/10
  Data Type Conversion9/1 -> PPEI_Hybrid_High_Voltage_Status/11
  Data Type Conversion10/1 -> PPEI_Hybrid_High_Voltage_Status/12
  Data Type Conversion11/1 -> PPEI_Hybrid_High_Voltage_Status/13
  Data Type Conversion12/1 -> PPEI_Hybrid_High_Voltage_Status/14
  Constant10/1 -> Data Type Conversion14/1
  Data Type Conversion14/1 -> PPEI_Hybrid_High_Voltage_Status/4

== system HIL_Testing_SW/TX/TX PTEI/Tx_Contactor_Msg/msg_0xCA ==
  busVltg : Inport  OutDataType=sfix(16)  OutScaling=2^0
  ContactorLine : Inport  Port=2  OutDataType=sfix(16)  OutScaling=2^0
  Trigger : TriggerPort  TriggerType=function-call
  Constant1 : Constant  Value=0  OutDataType=sfix(16)  OutScaling=2^0
  Constant2 : Constant  OutDataType=sfix(16)  OutScaling=2^0
  Constant3 : Constant  OutDataType=sfix(16)  OutScaling=2^0
  Constant4 : Constant  Value=.5  OutDataType=sfix(16)  OutScaling=2^0
  Data Type Conversion{1..3,7} (4 alike) : DataTypeConversion  OutDataType=fixdt(1, 16)  OutScaling=2^0
  Ground_1 : Ground
  Ground_2 : Ground
  HV_Battery_Information_1_PE : rtican/RTICAN Transmit (TX)   SystemSampleTime=-1  Reserved1=[]  Reserved2=[]  Reserved3=[]  Reserved4=[]  SfcnMessage=[]  Msg_Struct=[]  BoardTypeNo=[]  BoardNo=[]  ChannelNo=[]  Parameters=[]  DialogFcn=[]  UnitName=[]  Revision=[]  UnitValues=[]  DSProperties=struct('RTI',struct('Version',uint32(5),'BlockType',struct('isSLSource',uint8(1),'isSLSink',uint8(1),'isHWSource',uint8(0),'isHWSink',uint8(0),'isSetup',uint8(0),'isInline',uint8(1),'isNonInline',uint8(0),'isInterrupt',uint8(0),'isChannelwise',uint8(0)),'IOBoardType','RTICAN','UnitType','MESSAGE','Identifier','TX','DialogType','MSVC','BlockSet','RTICAN','SlaveProcessor','CAN'))  RTIBlockInterface=struct('InputPortsWidth',int32([1 1 1 1 1 1]),'InputPortsActive',[1 1 1 1 1 1],'InputPortsName',{{'HVBusNegToChsGVlt','HVBusPosToChsGVlt','HVBusNegToChsGVltV','HVBusPosToChsGVltV','HVBusNegToChsGVltM','HVBusPosToChsGVltM'}},'InputPortsDataType',{{'SS_DOUBLE','SS_DOUBLE','SS_DOUBLE','SS_DOUBLE','SS_DOUBLE','SS_DOUBLE'}},'OutputPortsWidth',int32(1),'OutputPortsActive',1,'OutputPortsName',{{['TX status']}},'DialogFcn','rtican_message_interface_gui','BlockDisplay',{{'','center'}},'IconTransparency','on','InitLevel',3,'BlockName',struct('Token',{{'HV_Battery_Information_1_PE'}}),'SampleTime',{{-1}},'TriggerPort',{{'none'}},'EnablePort',{{'none'}})  RTIBlockParameters=struct('BoardTypeNo',{{4302,'OFF',[]}},'BoardNo',{{1,'ON',[1 16]}},'ChannelNo',{{2,'ON',[1 4]}},'Parameters',{{struct('DataFileSupport',struct('DataFileSelectedMaster',1,'DataFileSelectedLocal',1,'DataFileName',['c:\data\databases\8.4.5 (140425)\globala - pe.dbc|'],'DataFileDate',{{{['24-Apr-2014 15:33:48']}}},'SelectedFile',['..\databases\8.4.5 (140425)\globala - pe.dbc'],'InterfaceFcn','rtican_dbc_file_parser'),'Options',struct('StatusSelected',1,'TimeSelected',0,'DeltaTimeSelected',0,'DelayTimeSelected',0,'DelayTimeTXCommandSelected',0,'EncodeSetUnusedBitsToOne',0,'EnableMsgLoopback',0,'TriggerPort',struct('Selected',0,'TriggerType',0),'EnablePortSelected',0,'SignalOnPortnameSelected',1,'UserCoding',struct('Selected',0,'InterfaceFile','UserEncodingFile','FcnName','UserEncodeFcn','InportSelected',0,'InportWidth',1,'OutportSelected',0,'OutportWidth',1),'TerminationMsg',struct('Selected',0,'Byte0_7','0'),'InitialMsg',struct('Selected',0,'Byte0_7','0')),'Message',struct('MsgOnBlocknameSelected',1,'MsgName','HV_Battery_Information_1_PE','MsgIdFormat',0,'MsgId',202,'MsgLength',3,'NumSignals',6,'SampleTime',-1,'StartTime',struct('Selected',0,'Value',0),'AutoRepeatTime',struct('Selected',0,'Value',0.1),'Timeout',struct('Selected',0,'Value',0.1),'DelayTime',struct('Selected',0,'Value',0.1),'Signal',struct('SgnName',{'HVBusNegToChsGVlt','HVBusPosToChsGVlt','HVBusNegToChsGVltV','HVBusPosToChsGVltV','HVBusNegToChsGVltM','HVBusPosToChsGVltM'},'SgnStartBit',{0,8,16,17,18,19},'SgnLength',{8,8,1,1,1,1},'SgnType',{0,0,0,0,0,0},'ModeValue',{-1,-1,-1,-1,-1,-1},'DataType',{0,0,0,0,0,0},'ByteLayout',{2,2,2,2,2,2},'Factor',{2,2,1,1,1,1},'Offset',{0,0,0,0,0,0},'SgnComment',{{''},{''},{''},{''},{''},{''}},'SgnUnit',{'volts','volts','','','',''},'Min',{0,0,0,0,0,0},'Max',{510,510,1,1,1,1},'SLDataType',{'SS_DOUBLE','SS_DOUBLE','SS_DOUBLE','SS_DOUBLE','SS_DOUBLE','SS_DOUBLE'}),'MsgIdNumFormat',0,'MsgComment',{{''}}),'Version',1.2,'general',struct('isFromLib',0)),'OFF',[]}},'GroupId',{{struct('Group',{{'RTICAN'}},'No',5,'Behavior',{{'NAMECHANGE'}},'BlockType',{{'SINK'}},'NameChangeFlag',0),'OFF',[]}},'SFcnRTICANMessage',{{struct('MsgType','TX','SFcnPortType','Scalar','MsgName','HV_Battery_Information_1_PE','MsgIdFormat','STD','MsgId',202,'MsgLength',3,'NumSignals',6,'SampleTime',-1,'StartTime',struct('Selected','no','Value',0),'AutoRepeatTime',struct('Selected','no','Value',0.1),'Timeout',struct('Selected','no','Value',0.1),'Signal',struct('SgnName',{'HVBusNegToChsGVlt','HVBusPosToChsGVlt','HVBusNegToChsGVltV','HVBusPosToChsGVltV','HVBusNegToChsGVltM','HVBusPosToChsGVltM'},'SgnStartBit',{0,8,16,17,18,19},'SgnLength',{8,8,1,1,1,1},'SgnType',{'standard','standard','standard','standard','standard','standard'},'ModeValue',{-1,-1,-1,-1,-1,-1},'DataType',{['unsigned int'],['unsigned int'],['unsigned int'],['unsigned int'],['unsigned int'],['unsigned int']},'ByteLayout',{['motorola back.'],['motorola back.'],['motorola back.'],['motorola back.'],['motorola back.'],['motorola back.']},'Factor',{2,2,1,1,1,1},'Offset',{0,0,0,0,0,0},'SLDataType',{'SS_DOUBLE','SS_DOUBLE','SS_DOUBLE','SS_DOUBLE','SS_DOUBLE','SS_DOUBLE'}),'StatusSelected','yes','TimeSelected','no','DeltaTimeSelected','no','DelayTimeSelected','no','DelayTimeTXCommandSelected','no','EncodeSetUnusedBitsToOne','no','EnableMsgLoopback','no','TriggerPort',struct('Selected','no','TriggerType',0),'EnablePortSelected','no','UserCoding',struct('Selected','no','InterfaceFile','UserEncodingFile','FcnName','UserEncodeFcn','InportSelected','no','InportWidth',1,'OutportSelected','no','OutportWidth',1),'TerminationMsg',struct('Selected','no','Byte0','0x00','Byte1','0x00','Byte2','0x00','Byte3','0x00','Byte4','0x00','Byte5','0x00','Byte6','0x00','Byte7','0x00'),'InitialMsg',struct('Selected','no','Byte0','0x00','Byte1','0x00','Byte2','0x00','Byte3','0x00','Byte4','0x00','Byte5','0x00','Byte6','0x00','Byte7','0x00'),'BoardType','DS4302','BoardNo',1,'ControllerNo',2),'OFF',[]}},'TLCFileName',{{'rtican_tx_message','OFF',[]}})  RTISFcnParameters=struct('SFcnRTICANMessage','struct','TLCFileName','char')  RTIBlockParaDefault=struct('BoardTypeNo',4302,'BoardNo',1,'ChannelNo',1,'Parameters',struct('DataFileSupport',struct('DataFileSelectedMaster',0,'DataFileSelectedLocal',0,'DataFileName','','DataFileDate','','SelectedFile',['<no file selected>']),'Options',struct('StatusSelected',1,'TimeSelected',1,'DeltaTimeSelected',1,'DelayTimeSelected',1,'DelayTimeTXCommandSelected',0,'EncodeSetUnusedBitsToOne',0,'EnableMsgLoopback',0,'TriggerPort',struct('Selected',0,'TriggerType','rising'),'EnablePortSelected',0,'SignalOnPortnameSelected',1,'UserCoding',struct('Selected',0,'InterfaceFile','UserEncodingFile','FcnName','UserEncodeFcn','InportSelected',0,'InportWidth',1,'OutportSelected',0,'OutportWidth',1),'TerminationMsg',struct('Selected',0,'Byte0_7','0'),'InitialMsg',struct('Selected',0,'Byte0_7','0')),'Message',struct('MsgOnBlocknameSelected',0,'MsgName',['TX Message'],'MsgIdFormat',0,'MsgId',100,'MsgLength',8,'NumSignals',1,'SampleTime',-1,'StartTime',struct('Selected',0,'Value',0),'AutoRepeatTime',struct('Selected',0,'Value',0.1),'Timeout',struct('Selected',0,'Value',0.1),'DelayTime',struct('Selected',0,'Value',0.1),'Signal',struct('SgnName',['TX signal'],'SgnStartBit',0,'SgnLength',8,'SgnType',0,'ModeValue',-1,'DataType',0,'SLDataType','SS_DOUBLE','ByteLayout',0,'Factor',1,'Offset',0,'Min',0,'Max',255,'SgnComment',{{}},'SgnUnit',''),'MsgIdNumFormat',0,'MsgComment',{{''}}),'Version',1.2,'general',struct('isFromLib',1)),'GroupId',struct('Group',{{'RTICAN'}},'No',1,'Behavior',{{'NAMECHANGE'}},'BlockType',{{'SINK'}},'NameChangeFlag',0),'SFcnRTICANMessage',struct('MsgType','TX','MsgName',['TX Message'],'MsgIdFormat','STD','MsgId',100,'MsgLength',2,'NumSignals',1,'SampleTime',-1,'StartTime',struct('Selected','no','Value',0),'AutoRepeatTime',struct('Selected','no','Value',0.1),'Timeout',struct('Selected','no','Value',0.1),'DelayTime',struct('Selected','no','Value',0.1),'Signal',struct('SgnName',['TX signal'],'SgnStartBit',0,'SgnLength',8,'SgnType','standard','ModeValue',-1,'DataType',['unsigned int'],'ByteLayout',['little endian'],'SLDataType','SS_DOUBLE','Factor',1,'Offset',0),'StatusSelected','yes','TimeSelected','yes','DeltaTimeSelected','yes','DelayTimeSelected','yes','EnablePortSelected','no','EnableMsgLoopback','no','DelayTimeTXCommandSelected','no','EncodeSetUnusedBitsToOne','no','UserCoding',struct('Selected','no','InterfaceFile','UserDecodingFile','FcnName','UserDecodeFcn','InportSelected','no','InportWidth',1,'OutportSelected','no','OutportWidth',1),'TerminationMsg',struct('Selected','no','Byte0','0x00','Byte1','0x00','Byte2','0x00','Byte3','0x00','Byte4','0x00','Byte5','0x00','Byte6','0x00','Byte7','0x00'),'InitialMsg',struct('Selected','no','Byte0','0x00','Byte1','0x00','Byte2','0x00','Byte3','0x00','Byte4','0x00','Byte5','0x00','Byte6','0x00','Byte7','0x00'),'TriggerPort',struct('Selected','no','TriggerType','rising'),'BoardType','DS4302','BoardNo',1,'ControllerNo',1,'SFcnPortType','Scalar'),'TLCFileName','rtican_tx_message')
      settings: AttributesFormatString=Group Id: RTICAN5\n
  Product : Product  OutDataType=sfix(16)  OutScaling=2^0  RndMeth=Zero
  Switch : Switch  Threshold=0.5  OutDataType=sfix(16)  OutScaling=2^0
  Terminator : Terminator
  wires:
  HV_Battery_Information_1_PE/1 -> Terminator/1
  Constant2/1 -> Data Type Conversion2/1
  Constant3/1 -> Data Type Conversion3/1
  ContactorLine/1 -> Switch/2
  Constant1/1 -> Switch/3
  busVltg/1 -> Product/1
  Constant4/1 -> Product/2
  Product/1 -> Switch/1
  Switch/1 -> Data Type Conversion7/1, Data Type Conversion1/1
  Ground_1/1 -> HV_Battery_Information_1_PE/3
  Ground_2/1 -> HV_Battery_Information_1_PE/4
  Data Type Conversion7/1 -> HV_Battery_Information_1_PE/1
  Data Type Conversion1/1 -> HV_Battery_Information_1_PE/2
  Data Type Conversion2/1 -> HV_Battery_Information_1_PE/5
  Data Type Conversion3/1 -> HV_Battery_Information_1_PE/6

== system HIL_Testing_SW/TX/Tx_Cycler/Send Ping/Trigger_1000ms ==
  Function-Call Generator : simulink/Ports & Subsystems/Function-Call Generator  sample_time=1  numberOfIterations=1
  Output Parameter : Outport  OutDataType=sfix(16)  OutScaling=2^0
  wires:
  Function-Call Generator/1 -> Output Parameter/1

== system HIL_Testing_SW/TX/Tx_Cycler/Send Ping/msg_0x1EO_Request_ABC ==
  note: 0x0140
  function : TriggerPort  TriggerType=function-call
  Constant8 : Constant  Value=320  OutDataType=sfix(16)  OutScaling=2^0
  Data Type Conversion7 : DataTypeConversion  OutDataType=fixdt(1, 16)  OutScaling=2^0
  Request_ABC : rtican/RTICAN Transmit (TX)   SystemSampleTime=-1  Reserved1=[]  Reserved2=[]  Reserved3=[]  Reserved4=[]  SfcnMessage=[]  Msg_Struct=[]  BoardTypeNo=[]  BoardNo=[]  ChannelNo=[]  Parameters=[]  DialogFcn=[]  UnitName=[]  Revision=[]  UnitValues=[]  DSProperties=struct('RTI',struct('Version',uint32(5),'BlockType',struct('isSLSource',uint8(1),'isSLSink',uint8(1),'isHWSource',uint8(0),'isHWSink',uint8(0),'isSetup',uint8(0),'isInline',uint8(1),'isNonInline',uint8(0),'isInterrupt',uint8(0),'isChannelwise',uint8(0)),'IOBoardType','RTICAN','UnitType','MESSAGE','Identifier','TX','DialogType','MSVC','BlockSet','RTICAN','SlaveProcessor','CAN'))  RTIBlockInterface=struct('InputPortsWidth',int32(1),'InputPortsActive',1,'InputPortsName',{{'Requested_CAN_ID_ABC'}},'InputPortsDataType',{{'SS_DOUBLE'}},'OutputPortsWidth',int32(1),'OutputPortsActive',1,'OutputPortsName',{{['TX status']}},'DialogFcn','rtican_message_interface_gui','BlockDisplay',{{'','center'}},'IconTransparency','on','InitLevel',3,'BlockName',struct('Token',{{'Request_ABC'}}),'SampleTime',{{-1}},'TriggerPort',{{'none'}},'EnablePort',{{'none'}})  RTIBlockParameters=struct('BoardTypeNo',{{2211,'OFF',[]}},'BoardNo',{{2,'ON',[1 16]}},'ChannelNo',{{1,'ON',[1 2]}},'Parameters',{{struct('DataFileSupport',struct('DataFileSelectedMaster',1,'DataFileSelectedLocal',1,'DataFileName','c:\data\testing\av900_dbc\av900_mod.dbc|','DataFileDate',{{{['16-Dec-2011 14:28:38']},{['10-May-2011 15:45:58']}}},'SelectedFile','av900_dbc\av900_mod.dbc','InterfaceFcn','rtican_dbc_file_parser'),'Options',struct('StatusSelected',1,'TimeSelected',0,'DeltaTimeSelected',0,'DelayTimeSelected',0,'DelayTimeTXCommandSelected',0,'EncodeSetUnusedBitsToOne',0,'EnableMsgLoopback',0,'TriggerPort',struct('Selected',0,'TriggerType',0),'EnablePortSelected',0,'SignalOnPortnameSelected',1,'UserCoding',struct('Selected',0,'InterfaceFile','UserEncodingFile','FcnName','UserEncodeFcn','InportSelected',0,'InportWidth',1,'OutportSelected',0,'OutportWidth',1),'TerminationMsg',struct('Selected',0,'Byte0_7','0'),'InitialMsg',struct('Selected',0,'Byte0_7','0')),'Message',struct('MsgOnBlocknameSelected',1,'MsgName','Request_ABC','MsgIdFormat',0,'MsgId',480,'MsgLength',2,'NumSignals',1,'SampleTime',-1,'StartTime',struct('Selected',0,'Value',0),'AutoRepeatTime',struct('Selected',0,'Value',0.1),'Timeout',struct('Selected',0,'Value',0.1),'DelayTime',struct('Selected',0,'Value',0.1),'Signal',struct('SgnName','Requested_CAN_ID_ABC','SgnStartBit',0,'SgnLength',16,'SgnType',0,'ModeValue',-1,'DataType',0,'ByteLayout',2,'Factor',1,'Offset',0,'SgnComment',{{''}},'SgnUnit','code','Min',0,'Max',65535,'SLDataType','SS_DOUBLE'),'MsgIdNumFormat',0,'MsgComment',{{''}}),'Version',1.2,'general',struct('isFromLib',0)),'OFF',[]}},'GroupId',{{struct('Group',{{'RTICAN'}},'No',6,'Behavior',{{'NAMECHANGE'}},'BlockType',{{'SINK'}},'NameChangeFlag',0),'OFF',[]}},'SFcnRTICANMessage',{{struct('MsgType','TX','SFcnPortType','Scalar','MsgName','Request_ABC','MsgIdFormat','STD','MsgId',480,'MsgLength',2,'NumSignals',1,'SampleTime',-1,'StartTime',struct('Selected','no','Value',0),'AutoRepeatTime',struct('Selected','no','Value',0.1),'Timeout',struct('Selected','no','Value',0.1),'Signal',struct('SgnName','Requested_CAN_ID_ABC','SgnStartBit',0,'SgnLength',16,'SgnType','standard','ModeValue',-1,'DataType',['unsigned int'],'ByteLayout',['motorola back.'],'Factor',1,'Offset',0,'SLDataType','SS_DOUBLE'),'StatusSelected','yes','TimeSelected','no','DeltaTimeSelected','no','DelayTimeSelected','no','DelayTimeTXCommandSelected','no','EncodeSetUnusedBitsToOne','no','EnableMsgLoopback','no','TriggerPort',struct('Selected','no','TriggerType',0),'EnablePortSelected','no','UserCoding',struct('Selected','no','InterfaceFile','UserEncodingFile','FcnName','UserEncodeFcn','InportSelected','no','InportWidth',1,'OutportSelected','no','OutportWidth',1),'TerminationMsg',struct('Selected','no','Byte0','0x00','Byte1','0x00','Byte2','0x00','Byte3','0x00','Byte4','0x00','Byte5','0x00','Byte6','0x00','Byte7','0x00'),'InitialMsg',struct('Selected','no','Byte0','0x00','Byte1','0x00','Byte2','0x00','Byte3','0x00','Byte4','0x00','Byte5','0x00','Byte6','0x00','Byte7','0x00'),'BoardType','DS2211','BoardNo',2,'ControllerNo',1),'OFF',[]}},'TLCFileName',{{'rtican_tx_message','OFF',[]}})  RTISFcnParameters=struct('SFcnRTICANMessage','struct','TLCFileName','char')  RTIBlockParaDefault=struct('BoardTypeNo',4302,'BoardNo',1,'ChannelNo',1,'Parameters',struct('DataFileSupport',struct('DataFileSelectedMaster',0,'DataFileSelectedLocal',0,'DataFileName','','DataFileDate','','SelectedFile',['<no file selected>']),'Options',struct('StatusSelected',1,'TimeSelected',1,'DeltaTimeSelected',1,'DelayTimeSelected',1,'DelayTimeTXCommandSelected',0,'EncodeSetUnusedBitsToOne',0,'EnableMsgLoopback',0,'TriggerPort',struct('Selected',0,'TriggerType','rising'),'EnablePortSelected',0,'SignalOnPortnameSelected',1,'UserCoding',struct('Selected',0,'InterfaceFile','UserEncodingFile','FcnName','UserEncodeFcn','InportSelected',0,'InportWidth',1,'OutportSelected',0,'OutportWidth',1),'TerminationMsg',struct('Selected',0,'Byte0_7','0'),'InitialMsg',struct('Selected',0,'Byte0_7','0')),'Message',struct('MsgOnBlocknameSelected',0,'MsgName',['TX Message'],'MsgIdFormat',0,'MsgId',100,'MsgLength',8,'NumSignals',1,'SampleTime',-1,'StartTime',struct('Selected',0,'Value',0),'AutoRepeatTime',struct('Selected',0,'Value',0.1),'Timeout',struct('Selected',0,'Value',0.1),'DelayTime',struct('Selected',0,'Value',0.1),'Signal',struct('SgnName',['TX signal'],'SgnStartBit',0,'SgnLength',8,'SgnType',0,'ModeValue',-1,'DataType',0,'SLDataType','SS_DOUBLE','ByteLayout',0,'Factor',1,'Offset',0,'Min',0,'Max',255,'SgnComment',{{}},'SgnUnit',''),'MsgIdNumFormat',0,'MsgComment',{{''}}),'Version',1.2,'general',struct('isFromLib',1)),'GroupId',struct('Group',{{'RTICAN'}},'No',1,'Behavior',{{'NAMECHANGE'}},'BlockType',{{'SINK'}},'NameChangeFlag',0),'SFcnRTICANMessage',struct('MsgType','TX','MsgName',['TX Message'],'MsgIdFormat','STD','MsgId',100,'MsgLength',2,'NumSignals',1,'SampleTime',-1,'StartTime',struct('Selected','no','Value',0),'AutoRepeatTime',struct('Selected','no','Value',0.1),'Timeout',struct('Selected','no','Value',0.1),'DelayTime',struct('Selected','no','Value',0.1),'Signal',struct('SgnName',['TX signal'],'SgnStartBit',0,'SgnLength',8,'SgnType','standard','ModeValue',-1,'DataType',['unsigned int'],'ByteLayout',['little endian'],'SLDataType','SS_DOUBLE','Factor',1,'Offset',0),'StatusSelected','yes','TimeSelected','yes','DeltaTimeSelected','yes','DelayTimeSelected','yes','EnablePortSelected','no','EnableMsgLoopback','no','DelayTimeTXCommandSelected','no','EncodeSetUnusedBitsToOne','no','UserCoding',struct('Selected','no','InterfaceFile','UserDecodingFile','FcnName','UserDecodeFcn','InportSelected','no','InportWidth',1,'OutportSelected','no','OutportWidth',1),'TerminationMsg',struct('Selected','no','Byte0','0x00','Byte1','0x00','Byte2','0x00','Byte3','0x00','Byte4','0x00','Byte5','0x00','Byte6','0x00','Byte7','0x00'),'InitialMsg',struct('Selected','no','Byte0','0x00','Byte1','0x00','Byte2','0x00','Byte3','0x00','Byte4','0x00','Byte5','0x00','Byte6','0x00','Byte7','0x00'),'TriggerPort',struct('Selected','no','TriggerType','rising'),'BoardType','DS4302','BoardNo',1,'ControllerNo',1,'SFcnPortType','Scalar'),'TLCFileName','rtican_tx_message')
      settings: AttributesFormatString=Group Id: RTICAN6\n
  Terminator : Terminator
  wires:
  Request_ABC/1 -> Terminator/1
  Constant8/1 -> Data Type Conversion7/1
  Data Type Conversion7/1 -> Request_ABC/1

== system HIL_Testing_SW/TX/Tx_Cycler/Subsystem/OurLatchReset ==
  U : Inport  OutDataType=fixdt(1, 16)  OutScaling=2^0
  Reset : Inport  Port=2  OutDataType=fixdt(1, 16)  OutScaling=2^0
  Logical Operator : Logic  Operator=NOT  AllPortsSameDT=off  OutDataTypeMode=boolean  LogicDataType=fixdt(0, 8)  OutDataTypeStr=boolean
  Logical Operator1 : Logic  Operator=OR  AllPortsSameDT=off  OutDataTypeMode=boolean  LogicDataType=fixdt(0, 8)  OutDataTypeStr=boolean
  Logical Operator2 : Logic  AllPortsSameDT=off  OutDataTypeMode=boolean  LogicDataType=fixdt(0, 8)  OutDataTypeStr=boolean
  Unit Delay : UnitDelay  SampleTime=-1
  Out1 : Outport  OutDataType=fixdt(1, 16)  OutScaling=2^0
  wires:
  Unit Delay/1 -> Logical Operator2/2
  Logical Operator1/1 -> Unit Delay/1, Out1/1
  U/1 -> Logical Operator1/1
  Logical Operator2/1 -> Logical Operator1/2
  Logical Operator/1 -> Logical Operator2/1
  Reset/1 -> Logical Operator/1
